simulink model "CIC"  (R2020b)
settings: Solver=VariableStepAuto  StartTime=0.0  StopTime=10000  RelTol=1e-3
settings Model: Creator=LYX  LastModifiedBy=LYX

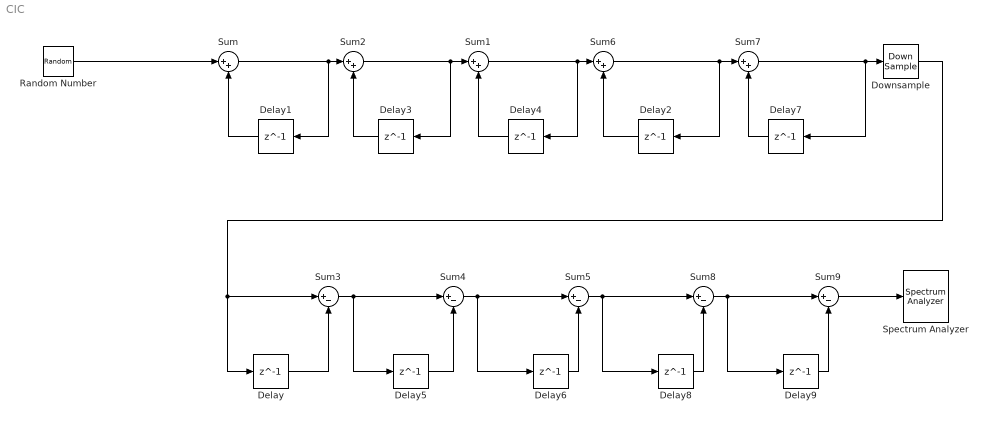
== system CIC ==
  Delay{,1..9} (10 alike) : Delay  DelayLength=1  InitialCondition=0
  Downsample : DownSample  N=8
  Random Number : RandomNumber  SampleTime=0.1
  Spectrum Analyzer : SpectrumAnalyzer
  Sum{,1..2,6..7} (5 alike) : Sum  Inputs=|++
  Sum{3..5,8..9} (5 alike) : Sum  Inputs=|+-
  wires:
  Sum/1 -> Sum2/1, Delay1/1
  Sum2/1 -> Delay3/1, Sum1/1
  Delay1/1 -> Sum/2
  Sum1/1 -> Sum6/1, Delay4/1
  Delay3/1 -> Sum2/2
  Delay4/1 -> Sum1/2
  Downsample/1 -> Delay/1, Sum3/1
  Sum3/1 -> Delay5/1, Sum4/1
  Sum4/1 -> Delay6/1, Sum5/1
  Delay/1 -> Sum3/2
  Delay5/1 -> Sum4/2
  Delay6/1 -> Sum5/2
  Sum6/1 -> Sum7/1, Delay2/1
  Delay2/1 -> Sum6/2
  Delay7/1 -> Sum7/2
  Sum7/1 -> Downsample/1, Delay7/1
  Sum5/1 -> Delay8/1, Sum8/1
  Delay8/1 -> Sum8/2
  Sum8/1 -> Delay9/1, Sum9/1
  Delay9/1 -> Sum9/2
  Sum9/1 -> Spectrum Analyzer/1
  Random Number/1 -> Sum/1
